simulink model "quad_control"  (R2014a)
settings: Solver=ode45  StartTime=0.0  StopTime=30  FixedStep=0.01  RelTol=1e-3
InitFcn:
  | % --- Inner loop gains --------
  | Kp_roll = 0.05;
  | Kp_pitch = 0.05;
  | Kp_yaw = 0.2;
  | 
  | Ki_roll = 0.002;
  | Ki_pitch = 0.002;
  | Ki_yaw = 0.1;
  | 
  | Kd_roll = 0.004;
  | Kd_pitch = 0.004;
  | Kd_yaw = 0.04;
  | % --------------------------
  | 
  | % --- Outer loop gains --------
  | Kp_altitude = 10;
  | Kp_pos_x = 10;
  | Kp_pos_y = 10;
  | 
  | Ki_altitude = 0.01;
  | Ki_pos_x = 5;
  | Ki_pos_y = 5;
  | 
  | Kd_altitude = 1;
  | Kd_pos_x = 5;
  | Kd_pos_y = 5;
  | % --------------------------
  | 
  | % --- Saturation limits --------
  | pos_upper_limit = 1;
  | pos_lower_limit = -1;
  | 
  | atit_upper_limit = 5;
  | atit_lower_limit = -5;
  | % --------------------------
  | 
  | global clientID;
  | clientID=-1;
libraries: simulink_extras x6
settings Model: Creator=kleber  LastModifiedBy=kleber

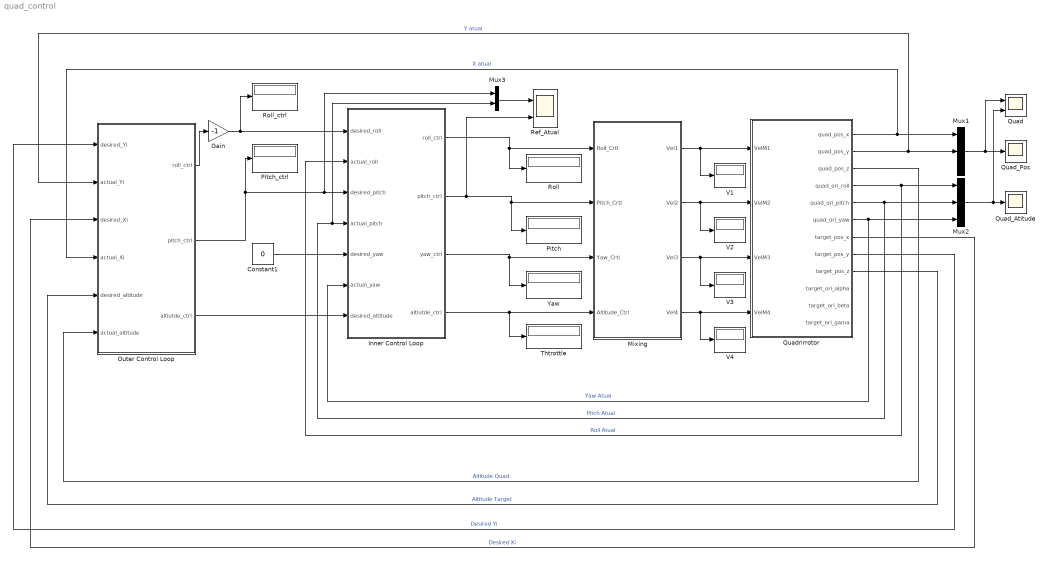
== system quad_control ==
  Constant1 : Constant  Value=0
  Gain : Gain  Gain=-1
  Inner Control Loop : Subsystem
  Mixing : Subsystem
  Mux1 : Mux  Inputs=3
  Mux2 : Mux  Inputs=3
  Mux3 : Mux  Inputs=2
  Outer Control Loop : Subsystem
  Pitch : Display
  Pitch_ctrl : Display
  Quad : Scope  NumInputPorts=2
      settings: ShowLegends=on  YMin=-0.2~-1.75  YMax=0.75~2.75  SaveName=ScopeData3
  Quad_Atitude : Scope
      settings: ShowLegends=on  TimeRange=5  YMin=-1.5  YMax=5.5
  Quad_Pos : Scope
      settings: ShowLegends=on  YMin=-0.09  YMax=0.09
  Quadrirrotor : Subsystem
  Ref_Atual : Scope  NumInputPorts=2
      settings: ShowLegends=on  YMin=-1.25~-0.05  YMax=1.25~0.055  SaveName=ScopeData2
  Roll : Display
  Roll_ctrl : Display
  Thtrottle : Display
  V{1..4} (4 alike) : Display
  Yaw : Display
  wires:
  Mux1/1 -> Quad/1, Quad_Pos/1
  Mux2/1 -> Quad/2, Quad_Atitude/1
  Quadrirrotor/5(quad_ori_pitch) -> Mux2/2, Mux3/2, Inner Control Loop/4(actual_pitch)  "Pitch Atual"
  Quadrirrotor/4(quad_ori_roll) -> Mux2/1, Inner Control Loop/2(actual_roll)  "Roll Atual"
  Quadrirrotor/1(quad_pos_x) -> Outer Control Loop/4(actual_Xi), Mux1/1  "X atual"
  Quadrirrotor/3(quad_pos_z) -> Outer Control Loop/6(actual_altitude)  "Altitude Quad"
  Quadrirrotor/6(quad_ori_yaw) -> Mux2/3, Inner Control Loop/6(actual_yaw)  "Yaw Atual"
  Mixing/1(Vel1) -> V1/1, Quadrirrotor/1(VelM1)
  Mixing/2(Vel2) -> Quadrirrotor/2(VelM2), V2/1
  Mixing/3(Vel3) -> Quadrirrotor/3(VelM3), V3/1
  Mixing/4(Vel4) -> Quadrirrotor/4(VelM4), V4/1
  Inner Control Loop/3(yaw_ctrl) -> Mixing/3(Yaw_Crtl), Yaw/1
  Inner Control Loop/1(roll_ctrl) -> Mixing/1(Roll_Crtl), Roll/1
  Inner Control Loop/4(altiutde_ctrl) -> Thtrottle/1, Mixing/4(Altitude_Ctrl)
  Inner Control Loop/2(pitch_ctrl) -> Ref_Atual/2, Pitch/1, Mixing/2(Pitch_Crtl)
  Outer Control Loop/3(altiutde_ctrl) -> Inner Control Loop/7(desired_altitude)
  Quadrirrotor/2(quad_pos_y) -> Outer Control Loop/2(actual_Yi), Mux1/2  "Y atual"
  Quadrirrotor/7(target_pos_x) -> Outer Control Loop/3(desired_Xi)  "Desired Xi"
  Quadrirrotor/8(target_pos_y) -> Outer Control Loop/1(desired_Yi)  "Desired Yi"
  Quadrirrotor/9(target_pos_z) -> Outer Control Loop/5(desired_altitude)  "Altitude Target"
  Constant1/1 -> Inner Control Loop/5(desired_yaw)
  Gain/1 -> Inner Control Loop/1(desired_roll), Roll_ctrl/1
  Mux3/1 -> Ref_Atual/1
  Outer Control Loop/1(roll_ctrl) -> Gain/1
  Outer Control Loop/2(pitch_ctrl) -> Pitch_ctrl/1, Mux3/1, Inner Control Loop/3(desired_pitch)

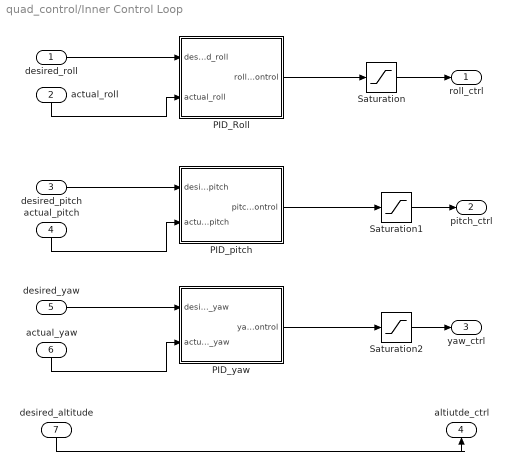
== system quad_control/Inner Control Loop ==
  desired_roll : Inport
  actual_roll : Inport  Port=2
  desired_pitch : Inport  Port=3
  actual_pitch : Inport  Port=4
  desired_yaw : Inport  Port=5
  actual_yaw : Inport  Port=6
  desired_altitude : Inport  Port=7
  PID_Roll : Subsystem
  PID_pitch : Subsystem
  PID_yaw : Subsystem
  Saturation : Saturate  UpperLimit=atit_upper_limit  LowerLimit=atit_lower_limit
  Saturation1 : Saturate  UpperLimit=atit_upper_limit  LowerLimit=atit_lower_limit
  Saturation2 : Saturate  UpperLimit=atit_upper_limit  LowerLimit=atit_lower_limit
  roll_ctrl : Outport
  pitch_ctrl : Outport  Port=2
  yaw_ctrl : Outport  Port=3
  altiutde_ctrl : Outport  Port=4
  wires:
  PID_yaw/1(yaw_control) -> Saturation2/1
  Saturation2/1 -> yaw_ctrl/1
  desired_yaw/1 -> PID_yaw/1(desired_yaw)
  actual_pitch/1 -> PID_pitch/2(actual_pitch)
  desired_altitude/1 -> altiutde_ctrl/1
  actual_yaw/1 -> PID_yaw/2(actual_yaw)
  actual_roll/1 -> PID_Roll/2(actual_roll)
  desired_roll/1 -> PID_Roll/1(desired_roll)
  Saturation/1 -> roll_ctrl/1
  Saturation1/1 -> pitch_ctrl/1
  desired_pitch/1 -> PID_pitch/1(desired_pitch)
  PID_Roll/1(roll_control) -> Saturation/1
  PID_pitch/1(pitch_control) -> Saturation1/1

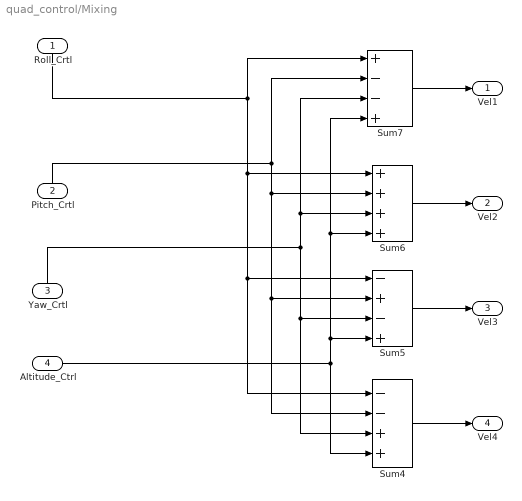
== system quad_control/Mixing ==
  Roll_Crtl : Inport
  Pitch_Crtl : Inport  Port=2
  Yaw_Crtl : Inport  Port=3
  Altitude_Ctrl : Inport  Port=4
  Sum4 : Sum  Inputs=--++
  Sum5 : Sum  Inputs=-+-+
  Sum6 : Sum  Inputs=++++
  Sum7 : Sum  Inputs=+--+
  Vel1 : Outport
  Vel2 : Outport  Port=2
  Vel3 : Outport  Port=3
  Vel4 : Outport  Port=4
  wires:
  Yaw_Crtl/1 -> Sum5/3, Sum4/3, Sum7/3, Sum6/3
  Roll_Crtl/1 -> Sum7/1, Sum6/1, Sum5/1, Sum4/1
  Pitch_Crtl/1 -> Sum5/2, Sum4/2, Sum6/2, Sum7/2
  Sum7/1 -> Vel1/1
  Sum6/1 -> Vel2/1
  Sum5/1 -> Vel3/1
  Sum4/1 -> Vel4/1
  Altitude_Ctrl/1 -> Sum7/4, Sum6/4, Sum5/4, Sum4/4

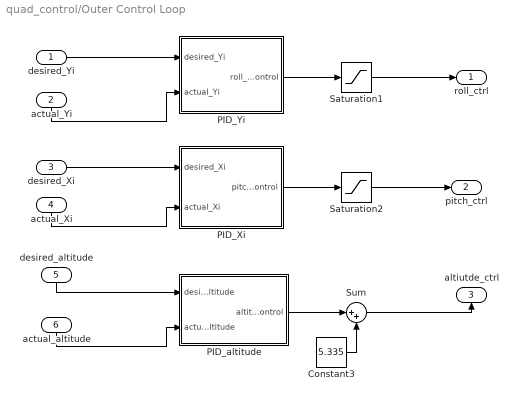
== system quad_control/Outer Control Loop ==
  desired_Yi : Inport
  actual_Yi : Inport  Port=2
  desired_Xi : Inport  Port=3
  actual_Xi : Inport  Port=4
  desired_altitude : Inport  Port=5
  actual_altitude : Inport  Port=6
  Constant3 : Constant  Value=5.335
  PID_Xi : Subsystem
  PID_Yi : Subsystem
  PID_altitude : Subsystem
  Saturation1 : Saturate  UpperLimit=pos_upper_limit  LowerLimit=pos_lower_limit
  Saturation2 : Saturate  UpperLimit=pos_upper_limit  LowerLimit=pos_lower_limit
  Sum : Sum  Inputs=|++
  roll_ctrl : Outport
  pitch_ctrl : Outport  Port=2
  altiutde_ctrl : Outport  Port=3
  wires:
  PID_Yi/1(roll_control) -> Saturation1/1
  PID_Xi/1(pitch_control) -> Saturation2/1
  Constant3/1 -> Sum/2
  desired_Yi/1 -> PID_Yi/1(desired_Yi)
  Sum/1 -> altiutde_ctrl/1
  desired_Xi/1 -> PID_Xi/1(desired_Xi)
  actual_Xi/1 -> PID_Xi/2(actual_Xi)
  desired_altitude/1 -> PID_altitude/1(desired_altitude)
  actual_altitude/1 -> PID_altitude/2(actual_altitude)
  actual_Yi/1 -> PID_Yi/2(actual_Yi)
  Saturation1/1 -> roll_ctrl/1
  Saturation2/1 -> pitch_ctrl/1
  PID_altitude/1(altitude_control) -> Sum/1

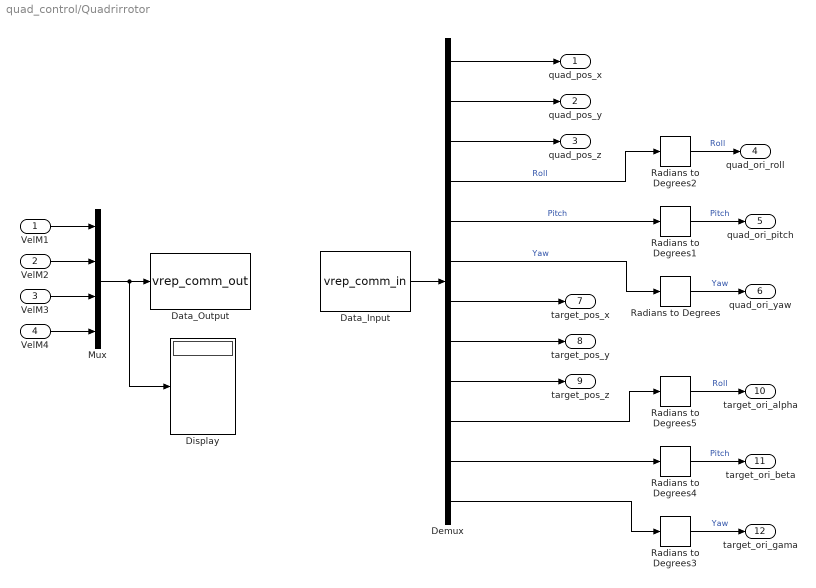
== system quad_control/Quadrirrotor ==
  VelM1 : Inport
  VelM2 : Inport  Port=2
  VelM3 : Inport  Port=3
  VelM4 : Inport  Port=4
  Data_Input : S-Function  FunctionName=vrep_comm_in  EnableBusSupport=off
  Data_Output : S-Function  FunctionName=vrep_comm_out  EnableBusSupport=off
  Demux : Demux  Outputs=12
  Display : Display
  Mux : Mux
  Radians to Degrees{,1..5} (6 alike) : simulink_extras/Transformations/Radians to Degrees
  quad_pos_x : Outport
  quad_pos_y : Outport  Port=2
  quad_pos_z : Outport  Port=3
  quad_ori_roll : Outport  Port=4
  quad_ori_pitch : Outport  Port=5
  quad_ori_yaw : Outport  Port=6
  target_pos_x : Outport  Port=7
  target_pos_y : Outport  Port=8
  target_pos_z : Outport  Port=9
  target_ori_alpha : Outport  Port=10
  target_ori_beta : Outport  Port=11
  target_ori_gama : Outport  Port=12
  wires:
  Mux/1 -> Display/1, Data_Output/1
  VelM1/1 -> Mux/1
  VelM2/1 -> Mux/2
  VelM3/1 -> Mux/3
  VelM4/1 -> Mux/4
  Demux/1 -> quad_pos_x/1
  Demux/2 -> quad_pos_y/1
  Demux/3 -> quad_pos_z/1
  Radians to Degrees2/1 -> quad_ori_roll/1  "Roll"
  Radians to Degrees1/1 -> quad_ori_pitch/1  "Pitch"
  Radians to Degrees/1 -> quad_ori_yaw/1  "Yaw"
  Demux/7 -> target_pos_x/1
  Demux/8 -> target_pos_y/1
  Demux/9 -> target_pos_z/1
  Demux/10 -> Radians to Degrees5/1
  Demux/11 -> Radians to Degrees4/1
  Demux/12 -> Radians to Degrees3/1
  Data_Input/1 -> Demux/1
  Demux/6 -> Radians to Degrees/1  "Yaw"
  Demux/5 -> Radians to Degrees1/1  "Pitch"
  Demux/4 -> Radians to Degrees2/1  "Roll"
  Radians to Degrees5/1 -> target_ori_alpha/1  "Roll"
  Radians to Degrees4/1 -> target_ori_beta/1  "Pitch"
  Radians to Degrees3/1 -> target_ori_gama/1  "Yaw"

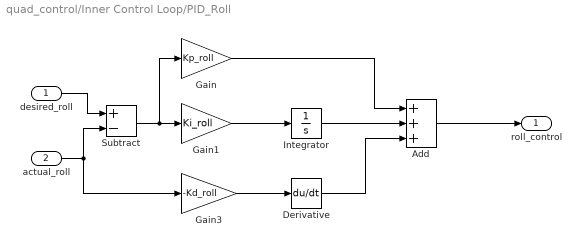
== system quad_control/Inner Control Loop/PID_Roll ==
  desired_roll : Inport
  actual_roll : Inport  Port=2
  Add : Sum  Inputs=+++
  Derivative : Derivative
  Gain : Gain  Gain=Kp_roll
  Gain1 : Gain  Gain=Ki_roll
  Gain3 : Gain  Gain=-Kd_roll
  Integrator : Integrator
  Subtract : Sum  Inputs=+-
  roll_control : Outport
  wires:
  Subtract/1 -> Gain1/1, Gain/1
  desired_roll/1 -> Subtract/1
  Add/1 -> roll_control/1
  Gain/1 -> Add/1
  Gain1/1 -> Integrator/1
  Gain3/1 -> Derivative/1
  actual_roll/1 -> Subtract/2, Gain3/1
  Integrator/1 -> Add/2
  Derivative/1 -> Add/3

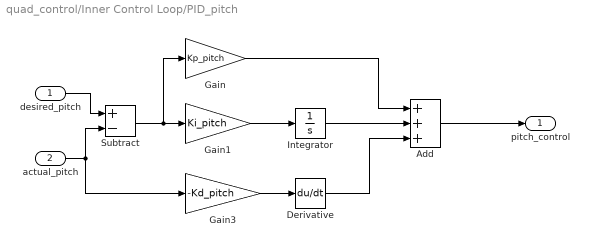
== system quad_control/Inner Control Loop/PID_pitch ==
  desired_pitch : Inport
  actual_pitch : Inport  Port=2
  Add : Sum  Inputs=+++
  Derivative : Derivative
  Gain : Gain  Gain=Kp_pitch
  Gain1 : Gain  Gain=Ki_pitch
  Gain3 : Gain  Gain=-Kd_pitch
  Integrator : Integrator
  Subtract : Sum  Inputs=+-
  pitch_control : Outport
  wires:
  Gain/1 -> Add/1
  Add/1 -> pitch_control/1
  desired_pitch/1 -> Subtract/1
  Subtract/1 -> Gain/1, Gain1/1
  Gain1/1 -> Integrator/1
  Gain3/1 -> Derivative/1
  actual_pitch/1 -> Gain3/1, Subtract/2
  Integrator/1 -> Add/2
  Derivative/1 -> Add/3

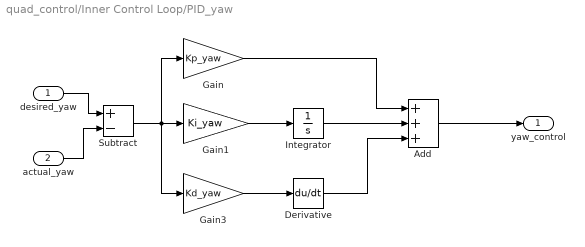
== system quad_control/Inner Control Loop/PID_yaw ==
  desired_yaw : Inport
  actual_yaw : Inport  Port=2
  Add : Sum  Inputs=+++
  Derivative : Derivative
  Gain : Gain  Gain=Kp_yaw
  Gain1 : Gain  Gain=Ki_yaw
  Gain3 : Gain  Gain=Kd_yaw
  Integrator : Integrator
  Subtract : Sum  Inputs=+-
  yaw_control : Outport
  wires:
  Gain3/1 -> Derivative/1
  Gain1/1 -> Integrator/1
  Subtract/1 -> Gain3/1, Gain1/1, Gain/1
  desired_yaw/1 -> Subtract/1
  Add/1 -> yaw_control/1
  Gain/1 -> Add/1
  actual_yaw/1 -> Subtract/2
  Derivative/1 -> Add/3
  Integrator/1 -> Add/2

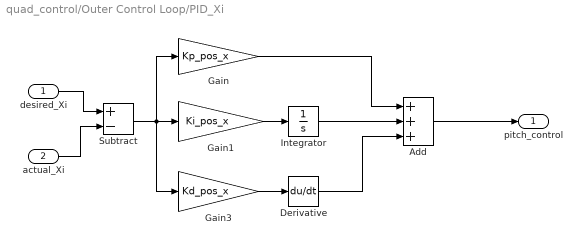
== system quad_control/Outer Control Loop/PID_Xi ==
  desired_Xi : Inport
  actual_Xi : Inport  Port=2
  Add : Sum  Inputs=+++
  Derivative : Derivative
  Gain : Gain  Gain=Kp_pos_x
  Gain1 : Gain  Gain=Ki_pos_x
  Gain3 : Gain  Gain=Kd_pos_x
  Integrator : Integrator
  Subtract : Sum  Inputs=+-
  pitch_control : Outport
  wires:
  Gain3/1 -> Derivative/1
  Gain1/1 -> Integrator/1
  Gain/1 -> Add/1
  Add/1 -> pitch_control/1
  desired_Xi/1 -> Subtract/1
  Subtract/1 -> Gain/1, Gain1/1, Gain3/1
  actual_Xi/1 -> Subtract/2
  Integrator/1 -> Add/2
  Derivative/1 -> Add/3

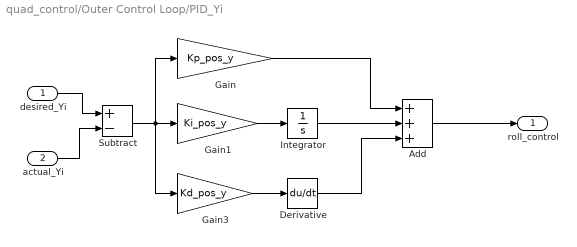
== system quad_control/Outer Control Loop/PID_Yi ==
  desired_Yi : Inport
  actual_Yi : Inport  Port=2
  Add : Sum  Inputs=+++
  Derivative : Derivative
  Gain : Gain  Gain=Kp_pos_y
  Gain1 : Gain  Gain=Ki_pos_y
  Gain3 : Gain  Gain=Kd_pos_y
  Integrator : Integrator
  Subtract : Sum  Inputs=+-
  roll_control : Outport
  wires:
  Gain3/1 -> Derivative/1
  Gain1/1 -> Integrator/1
  Subtract/1 -> Gain3/1, Gain1/1, Gain/1
  desired_Yi/1 -> Subtract/1
  Add/1 -> roll_control/1
  Gain/1 -> Add/1
  actual_Yi/1 -> Subtract/2
  Integrator/1 -> Add/2
  Derivative/1 -> Add/3

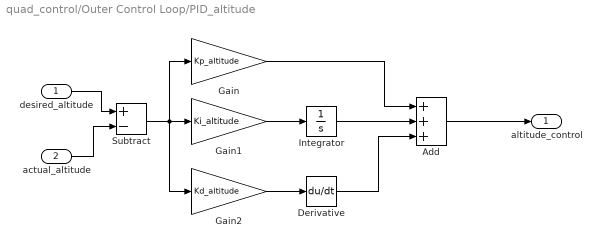
== system quad_control/Outer Control Loop/PID_altitude ==
  desired_altitude : Inport
  actual_altitude : Inport  Port=2
  Add : Sum  Inputs=+++
  Derivative : Derivative
  Gain : Gain  Gain=Kp_altitude
  Gain1 : Gain  Gain=Ki_altitude
  Gain2 : Gain  Gain=Kd_altitude
  Integrator : Integrator
  Subtract : Sum  Inputs=+-
  altitude_control : Outport
  wires:
  Gain2/1 -> Derivative/1
  Gain1/1 -> Integrator/1
  Gain/1 -> Add/1
  Add/1 -> altitude_control/1
  actual_altitude/1 -> Subtract/2
  desired_altitude/1 -> Subtract/1
  Subtract/1 -> Gain/1, Gain1/1, Gain2/1
  Integrator/1 -> Add/2
  Derivative/1 -> Add/3
